simulink model "CasaFarmaceutica"  (R2023b)
settings: Solver=VariableStepAuto  StartTime=0.0  StopTime=16  RelTol=1e-3
(part 2 of 2)

== matlab function CasaFarmaceutica/media ==
  data: u input; y output
function y = media(u)

y = mean(u);

== matlab function CasaFarmaceutica/media2 ==
  data: u input; y output
function y = media(u)

y = mean(u);

== matlab function CasaFarmaceutica/media3 ==
  data: u input; y output
function y = media(u)

y = mean(u);

== matlab function CasaFarmaceutica/media4 ==
  data: u input; y output
function y = media(u)

y = mean(u);

== matlab function CasaFarmaceutica/media1 ==
  data: u input; y output
function y = media(u)

y = mean(u);
